simulink subsystem "PvtSubSys_LONC"  (R2020b)
settings: Solver=VariableStepAuto  StartTime=0.0  StopTime=10.0  RelTol=1e-3
undefined symbols (not defined in the file): P_Global_TireRadius_m, P_Global_Weight_N, P_LongCtrl_AxvRoadSlopeThrd, P_LongCtrl_SlideFlagEnable, P_LongCtrl_TotWheelTrqRatio, P_LongCtrl_VLC_fRollCoef, P_LongCtrl_VLC_WindArea, P_LongCtrl_VLCaccelMinHoldXAxis, P_LongCtrl_VLCaccelMinHoldYAxis, P_LongCtrl_VLCaccelMinSlidHoldXAxis, P_LongCtrl_VLCaccelMinSlidHoldYAxis, P_LongCtrl_VLCaDiffCharCoefKiEnableXAxis, P_LongCtrl_VLCaDiffCharCoefKiXAxis, P_LongCtrl_VLCaDtThresUpdateTorq, P_LongCtrl_VLCaXCDeadZoneProp_Y, P_LongCtrl_VLCaxCtrlDevDeadZoneChar_Y, P_LongCtrl_VLCaxCtrlDevEC2DCMax, P_LongCtrl_VLCaxCtrlDevFastQuitDCMode, P_LongCtrl_VLCaxCtrlDevThresAddEC2DCCharYAxis, P_LongCtrl_VLCaxCtrlDevTresAddDC2ECYAxis, P_LongCtrl_VLCaxDtCharAxCtrlDevTresAddDC2ECXAxis, P_LongCtrl_VLCaxDtCharAxCtrlDevTresAddEC2DCXAxis, P_LongCtrl_VLCAxTarDtThreEnableI, P_LongCtrl_VLCaxvRoadSlopeDC4CharXAxis, P_LongCtrl_VLCaxvRoadSlopeDC4CharYAxis, P_LongCtrl_VLCAxvTracMinDC1FullFillXAxis, P_LongCtrl_VLCAxvTracMinDC1FullFillYAxis, P_LongCtrl_VLCcoefFXAxis, P_LongCtrl_VLCcoefFYAxis, P_LongCtrl_VLCcoefIFadeOut1Calc, P_LongCtrl_VLCcoefIFadeOut1Condition, P_LongCtrl_VLCcoefIFadeOut2Calc, P_LongCtrl_VLCcoefIFadeOut2Condition, P_LongCtrl_VLCcoefIFadeOut3Calc, P_LongCtrl_VLCcoefIFadeOut3Condition, P_LongCtrl_VLCcoefKiDiffDtEnlargeYAxis, P_LongCtrl_VLCcoefKiEnableYAxis, P_LongCtrl_VLCcoefKiEnlargeADiffYAxis, P_LongCtrl_VLCcoefPIYAxis, P_LongCtrl_VLCCounterAxvTracMinTimeout, P_LongCtrl_VLCCounterDC2ECTorqDelay, P_LongCtrl_VLCCounterDrvOff2EC, P_LongCtrl_VLCdaxTarEC2DCMax, P_LongCtrl_VLCdiffDtCharCoefKiEnlargeXAxis, P_LongCtrl_VLCdriveOffAxUpLimXAxix, P_LongCtrl_VLCdriveOffAxUpLimYAxix, P_LongCtrl_VLCDtAxvRef2UpperBandDC5, P_LongCtrl_VLCengEfficientCharYAxis, P_LongCtrl_VLCengInverseEfficientYAxis, P_LongCtrl_VLCIACompensionNeg, P_LongCtrl_VLCIACompensionPos, P_LongCtrl_VLCjerkHoldXAxis, P_LongCtrl_VLCjerkHoldYAxis, P_LongCtrl_VLCjerkSlidHoldXAxis, P_LongCtrl_VLCjerkSlidHoldYAxis, P_LongCtrl_VLCki, P_LongCtrl_VLCkp, P_LongCtrl_VLCks, P_LongCtrl_VLCLowerJerkCounterDrvOff2EC, P_LongCtrl_VLCMaRatioCharMaYAxis ... (+12)
libraries: simulink x34
(part 2 of 3)

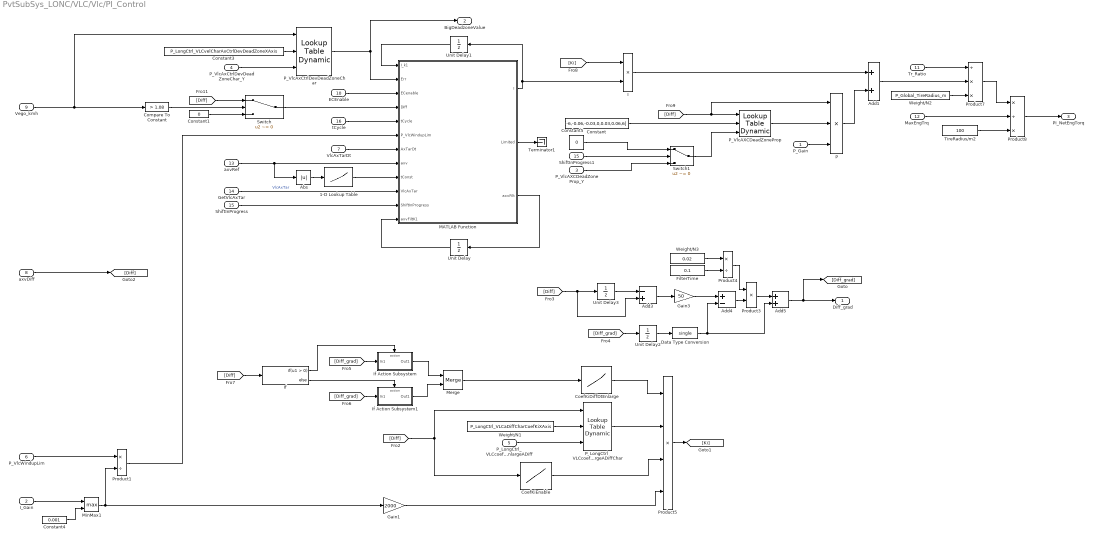
== system PvtSubSys_LONC/VLC/Vlc/PI_Control ==
  P_Gain : Inport
  I_Gain : Inport  Port=2
  P_VlcAXCDeadZoneProp_Y : Inport  Port=3
  P_VlcAxCtrlDevDeadZoneChar_Y : Inport  Port=4
  P_LongCtrl_VLCcoefKiEnlargeADiff : Inport  Port=5
  P_VlcWindupLim : Inport  Port=6
  VlcAxTarDt : Inport  Port=7
  axvDiff : Inport  Port=8
  Vego_kmh : Inport  Port=9
  ECEnable : Inport  Port=10
  Tr_Ratio : Inport  Port=11
  MaxEngTrq : Inport  Port=12
  axvRef : Inport  Port=13
  GetVlcAxTar : Inport  Port=14
  ShiftInProgress : Inport  Port=15
  tCycle : Inport  Port=16
  1-D Lookup Table : Lookup_n-D  NumberOfTableDimensions=1  BreakpointsForDimension1=[0,0.01,0.05,0.1,0.2,0.5]  Table=[0.02,0.06,0.1,0.2,0.3,0.3]  ExtrapMethod=Clip  UseLastTableValue=on  InternalRulePriority=Speed  RndMeth=Simplest  InputSameDT=on
  Abs : Abs
  Add1 : Sum
  Add3 : Sum  Inputs=-+
  Add4 : Sum  Inputs=+-  AccumDataTypeStr=single
  Add5 : Sum  AccumDataTypeStr=single
  CoefKiDiffDtEnlarge : Lookup_n-D  NumberOfTableDimensions=1  BreakpointsForDimension1=P_LongCtrl_VLCdiffDtCharCoefKiEnlargeXAxis  Table=P_LongCtrl_VLCcoefKiDiffDtEnlargeYAxis  ExtrapMethod=Clip  UseLastTableValue=on  RndMeth=Simplest  InputSameDT=on
  CoefKiEnable : Lookup_n-D  NumberOfTableDimensions=1  BreakpointsForDimension1=P_LongCtrl_VLCaDiffCharCoefKiEnableXAxis  Table=P_LongCtrl_VLCcoefKiEnableYAxis  ExtrapMethod=Clip  UseLastTableValue=on  RndMeth=Simplest  InputSameDT=on
  Compare To Constant : simulink/Logic and Bit Operations/Compare To Constant  relop=>  const=1.08  OutDataTypeStr=boolean
  Constant : Constant  Value=[-6,-0.06,-0.03,0,0.03,0.06,6]  OutDataTypeStr=single
  Constant1 : Constant  Value=0  OutDataTypeStr=single
  Constant3 : Constant  Description="0   36   72  108  120"  Value=P_LongCtrl_VLCvelCharAxCtrlDevDeadZoneXAxis  OutDataTypeStr=single
      settings: AttributesFormatString=%<Description>
  Constant4 : Constant  Value=0.001  OutDataTypeStr=single
  Constant5 : Constant  Value=0  OutDataTypeStr=single
  Data Type Conversion : DataTypeConversion  OutDataTypeStr=single
  FilterTime : Constant  Value=0.1  OutDataTypeStr=single
  Gain1 : Gain  Gain=2000
  Gain3 : Gain  Gain=50
  I : Product  RndMeth=Zero
  If : If
  If Action Subsystem : Subsystem  TreatAsAtomicUnit=on
  If Action Subsystem1 : Subsystem  TreatAsAtomicUnit=on
  MATLAB Function : MATLAB Function  TreatAsAtomicUnit=on
  Merge : Merge
  MinMax1 : MinMax  Function=max  Inputs=2
  P : Product  Inputs=3  RndMeth=Zero
  P_LongCtrl_VLCcoefKiEnlargeADiffChar : simulink/Lookup Tables/Lookup Table Dynamic  LookUpMeth=Interpolation-Use End Values  OutDataType=fixdt('single')  OutScaling=[]  OutputDataTypeScalingMode=Specify via dialog  OutDataTypeStr=single  DoSatur=off
  P_VlcAXCDeadZoneProp : simulink/Lookup Tables/Lookup Table Dynamic  LookUpMeth=Interpolation-Use End Values  OutDataType=fixdt('single')  OutScaling=[]  OutputDataTypeScalingMode=Specify via dialog  OutDataTypeStr=single  DoSatur=off
  P_VlcAxCtrlDevDeadZoneChar : simulink/Lookup Tables/Lookup Table Dynamic  LookUpMeth=Interpolation-Use End Values  OutDataType=fixdt('single')  OutScaling=[]  OutputDataTypeScalingMode=Specify via dialog  OutDataTypeStr=single  DoSatur=off
  Product1 : Product  Inputs=*/  RndMeth=Zero
  Product3 : Product  Inputs=**  RndMeth=Zero
  Product4 : Product  Inputs=*/  RndMeth=Zero
  Product5 : Product  Inputs=4  RndMeth=Zero
  Product7 : Product  Inputs=/**  RndMeth=Zero
  Product8 : Product  Inputs=*/*  RndMeth=Zero
  ShiftInProgress1 : InportShadow  Port=15
  Switch : Switch  Criteria=u2 ~= 0  Threshold=1.08
  Switch1 : Switch  Criteria=u2 ~= 0
  Terminator1 : Terminator
  TireRadius/m2 : Constant  Value=100  OutDataTypeStr=single
  Unit Delay : UnitDelay  SampleTime=-1  HasFrameUpgradeWarning=on
  Unit Delay1 : UnitDelay  SampleTime=-1  HasFrameUpgradeWarning=on
  Unit Delay2 : UnitDelay  InitialCondition=single(0)  SampleTime=-1  HasFrameUpgradeWarning=on
  Unit Delay3 : UnitDelay  SampleTime=-1  HasFrameUpgradeWarning=on
  Weight/N1 : Constant  Description="-2.5          -2        -0.4       -0.17        -0.1           0        0.15        0.25         0.6           3         3.5"  Value=P_LongCtrl_VLCaDiffCharCoefKiXAxis  OutDataTypeStr=single
      settings: AttributesFormatString=%<Description>
  Weight/N2 : Constant  Value=P_Global_TireRadius_m
  Weight/N3 : Constant  Value=0.02  OutDataTypeStr=single
  Diff_grad : Outport
  BigDeadzoneValue : Outport  Port=2
  PI_NetEngTorq : Outport  Port=3
  wires:
  Data Type Conversion/1 -> Add4/2, Add5/2
  Switch1/1 -> P_VlcAXCDeadZoneProp/3
  Constant5/1 -> Switch1/1
  ShiftInProgress1/1 -> Switch1/2
  Unit Delay/1 -> MATLAB Function/12(axvFiltK1)
  GetVlcAxTar/1 -> MATLAB Function/10(VlcAxTar)  "VlcAxTar"
  axvRef/1 -> Abs/1, MATLAB Function/8(axv)
  ShiftInProgress/1 -> MATLAB Function/11(ShiftInProgress)
  Abs/1 -> 1-D Lookup Table/1
  1-D Lookup Table/1 -> MATLAB Function/9(tConst)
  I_Gain/1 -> MinMax1/1
  Constant4/1 -> MinMax1/2
  axvDiff/1 -> [Diff]
  MATLAB Function/2(Limited) -> Terminator1/1
  Gain1/1 -> Product5/4
  Constant/1 -> P_VlcAXCDeadZoneProp/2
  MATLAB Function/3(axvFilt) -> Unit Delay/1
  Product1/1 -> MATLAB Function/6(P_VlcWindupLim)
  MinMax1/1 -> Product1/2, Gain1/1
  VlcAxTarDt/1 -> MATLAB Function/7(AxTarDt)
  P_VlcWindupLim/1 -> Product1/1
  I/1 -> Add1/1
  P_LongCtrl_VLCcoefKiEnlargeADiff/1 -> P_LongCtrl_VLCcoefKiEnlargeADiffChar/3
  Weight/N1/1 -> P_LongCtrl_VLCcoefKiEnlargeADiffChar/2
  Add1/1 -> Product7/2
  Product8/1 -> PI_NetEngTorq/1
  Weight/N2/1 -> Product7/3
  Tr_Ratio/1 -> Product7/1
  Product7/1 -> Product8/1
  MaxEngTrq/1 -> Product8/2
  TireRadius/m2/1 -> Product8/3
  P_VlcAxCtrlDevDeadZoneChar/1 -> MATLAB Function/2(Err), BigDeadzoneValue/1
  P_VlcAxCtrlDevDeadZoneChar_Y/1 -> P_VlcAxCtrlDevDeadZoneChar/3
  Constant3/1 -> P_VlcAxCtrlDevDeadZoneChar/2
  Unit Delay1/1 -> MATLAB Function/1(I_k1)
  ECEnable/1 -> MATLAB Function/3(ECenable)
  Switch/1 -> MATLAB Function/4(Diff)
  tCycle/1 -> MATLAB Function/5(tCycle)
  P_VlcAXCDeadZoneProp_Y/1 -> Switch1/3
  P_VlcAXCDeadZoneProp/1 -> P/2
  MATLAB Function/1(I) -> I/2, Unit Delay1/1
  [Diff] -> P_VlcAXCDeadZoneProp/1, P/1
  Product5/1 -> [Ki]
  CoefKiEnable/1 -> Product5/3
  P_LongCtrl_VLCcoefKiEnlargeADiffChar/1 -> Product5/2
  CoefKiDiffDtEnlarge/1 -> Product5/1
  [Diff] -> CoefKiEnable/1, P_LongCtrl_VLCcoefKiEnlargeADiffChar/1
  FilterTime/1 -> Product4/2
  Product4/1 -> Product3/1
  Weight/N3/1 -> Product4/1
  [Diff] -> If/1
  Merge/1 -> CoefKiDiffDtEnlarge/1
  If Action Subsystem1/1(Out1) -> Merge/2
  If Action Subsystem/1(Out1) -> Merge/1
  [Diff_grad] -> If Action Subsystem1/1(In1)
  [Diff_grad] -> If Action Subsystem/1(In1)
  If/2 -> If Action Subsystem1/Action
  If/1 -> If Action Subsystem/Action
  [Diff] -> Add3/2, Unit Delay3/1
  Gain3/1 -> Add4/1
  Add5/1 -> Diff_grad/1, [Diff_grad]
  Product3/1 -> Add5/1
  Add4/1 -> Product3/2
  Add3/1 -> Gain3/1
  Unit Delay2/1 -> Data Type Conversion/1
  [Diff_grad] -> Unit Delay2/1
  Unit Delay3/1 -> Add3/1
  Constant1/1 -> Switch/3
  Vego_kmh/1 -> P_VlcAxCtrlDevDeadZoneChar/1, Compare To Constant/1
  [Diff] -> Switch/1
  [Ki] -> I/1
  P/1 -> Add1/2
  P_Gain/1 -> P/3
  Compare To Constant/1 -> Switch/2

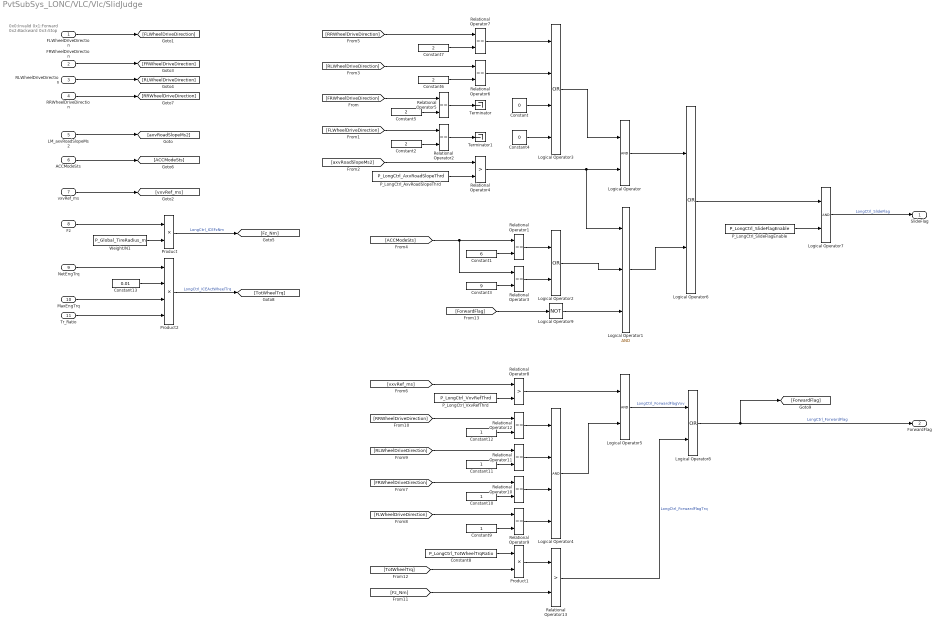
== system PvtSubSys_LONC/VLC/Vlc/SlidJudge ==
  note: 0x0:Invalid
      | 0x1:Forward
      | 0x2:Backward
      | 0x3:Stop
  FLWheelDriveDirection : Inport
  FRWheelDriveDirection : Inport  Port=2
  RLWheelDriveDirection : Inport  Port=3
  RRWheelDriveDirection : Inport  Port=4
  LM_axvRoadSlopeMs2 : Inport  Port=5
  ACCModeSts : Inport  Port=6
  vxvRef_ms : Inport  Port=7
  Fz : Inport  Port=8
  NetEngTrq : Inport  Port=9
  MaxEngTrq : Inport  Port=10
  Tr_Ratio : Inport  Port=11
  Constant : Constant  Value=0  OutDataTypeStr=boolean
  Constant1 : Constant  Value=6
  Constant{9..12} (4 alike) : Constant
  Constant13 : Constant  Value=0.01
  Constant{2,5..7} (4 alike) : Constant  Value=2
  Constant3 : Constant  Value=9
  Constant4 : Constant  Value=0  OutDataTypeStr=boolean
  Constant8 : Constant  Value=P_LongCtrl_TotWheelTrqRatio
  Logical Operator : Logic  AllPortsSameDT=off  OutDataTypeStr=boolean
  Logical Operator1 : Logic  Inputs=3  AllPortsSameDT=off  OutDataTypeStr=boolean
  Logical Operator2 : Logic  Operator=OR  AllPortsSameDT=off  OutDataTypeStr=boolean
  Logical Operator3 : Logic  Operator=OR  Inputs=4  AllPortsSameDT=off  OutDataTypeStr=boolean
  Logical Operator4 : Logic  Inputs=4  AllPortsSameDT=off  OutDataTypeStr=boolean
  Logical Operator5 : Logic  AllPortsSameDT=off  OutDataTypeStr=boolean
  Logical Operator6 : Logic  Operator=OR  AllPortsSameDT=off  OutDataTypeStr=boolean
  Logical Operator7 : Logic  AllPortsSameDT=off  OutDataTypeStr=boolean
  Logical Operator8 : Logic  Operator=OR  AllPortsSameDT=off  OutDataTypeStr=boolean
  Logical Operator9 : Logic  Operator=NOT  AllPortsSameDT=off  OutDataTypeStr=boolean
  P_LongCtrl_AxvRoadSlopeThrd : Constant  Description=0.1  Value=P_LongCtrl_AxvRoadSlopeThrd
      settings: AttributesFormatString=%<Description>
  P_LongCtrl_SlideFlagEnable : Constant  Description=0  Value=P_LongCtrl_SlideFlagEnable
      settings: AttributesFormatString=%<Description>
  P_LongCtrl_VxvRefThrd : Constant  Description=0.1  Value=P_LongCtrl_VxvRefThrd
      settings: AttributesFormatString=%<Description>
  Product : Product
  Product1 : Product
  Product2 : Product  Inputs=4
  Relational Operator{1..3,5..7,9..12} (10 alike) : RelationalOperator  Operator===  OutDataTypeStr=boolean  RndMeth=Simplest
  Relational Operator13 : RelationalOperator  Operator=>  OutDataTypeStr=boolean  RndMeth=Simplest
  Relational Operator4 : RelationalOperator  Operator=>  OutDataTypeStr=boolean  RndMeth=Simplest
  Relational Operator8 : RelationalOperator  Operator=>  OutDataTypeStr=boolean  RndMeth=Simplest
  Terminator : Terminator
  Terminator1 : Terminator
  Weight/N1 : Constant  Value=P_Global_TireRadius_m
  SlideFlag : Outport
  ForwardFlag : Outport  Port=2
  wires:
  Constant2/1 -> Relational Operator2/2
  FRWheelDriveDirection/1 -> [FRWheelDriveDirection]
  RLWheelDriveDirection/1 -> [RLWheelDriveDirection]
  RRWheelDriveDirection/1 -> [RRWheelDriveDirection]
  LM_axvRoadSlopeMs2/1 -> [axvRoadSlopeMs2]
  P_LongCtrl_AxvRoadSlopeThrd/1 -> Relational Operator4/2
  Relational Operator2/1 -> Terminator1/1
  Relational Operator4/1 -> Logical Operator1/1, Logical Operator/2
  FLWheelDriveDirection/1 -> [FLWheelDriveDirection]
  [FLWheelDriveDirection] -> Relational Operator2/1
  [axvRoadSlopeMs2] -> Relational Operator4/1
  ACCModeSts/1 -> [ACCModeSts]
  [ACCModeSts] -> Relational Operator3/1, Relational Operator1/1
  Constant1/1 -> Relational Operator1/2
  Constant3/1 -> Relational Operator3/2
  Relational Operator1/1 -> Logical Operator2/1
  Relational Operator3/1 -> Logical Operator2/2
  Logical Operator2/1 -> Logical Operator1/2
  Logical Operator1/1 -> Logical Operator6/2
  Logical Operator/1 -> Logical Operator6/1
  Relational Operator5/1 -> Terminator/1
  Constant5/1 -> Relational Operator5/2
  Constant6/1 -> Relational Operator6/2
  Relational Operator6/1 -> Logical Operator3/2
  Relational Operator7/1 -> Logical Operator3/1
  Constant7/1 -> Relational Operator7/2
  [RRWheelDriveDirection] -> Relational Operator7/1
  [RLWheelDriveDirection] -> Relational Operator6/1
  [FRWheelDriveDirection] -> Relational Operator5/1
  Logical Operator3/1 -> Logical Operator/1
  vxvRef_ms/1 -> [vxvRef_ms]
  [vxvRef_ms] -> Relational Operator8/1
  P_LongCtrl_VxvRefThrd/1 -> Relational Operator8/2
  [FRWheelDriveDirection] -> Relational Operator10/1
  [RLWheelDriveDirection] -> Relational Operator11/1
  [RRWheelDriveDirection] -> Relational Operator12/1
  Constant12/1 -> Relational Operator12/2
  Relational Operator12/1 -> Logical Operator4/1
  Relational Operator11/1 -> Logical Operator4/2
  Constant11/1 -> Relational Operator11/2
  Constant10/1 -> Relational Operator10/2
  Relational Operator10/1 -> Logical Operator4/3
  [FLWheelDriveDirection] -> Relational Operator9/1
  Relational Operator9/1 -> Logical Operator4/4
  Constant9/1 -> Relational Operator9/2
  Relational Operator8/1 -> Logical Operator5/1
  Logical Operator4/1 -> Logical Operator5/2
  Logical Operator5/1 -> Logical Operator8/1  "LongCtrl_ForwardFlagVxv"
  Logical Operator6/1 -> Logical Operator7/1
  Logical Operator7/1 -> SlideFlag/1  "LongCtrl_SlideFlag"
  P_LongCtrl_SlideFlagEnable/1 -> Logical Operator7/2
  Constant/1 -> Logical Operator3/3
  Constant4/1 -> Logical Operator3/4
  Fz/1 -> Product/1
  Weight/N1/1 -> Product/2
  Product/1 -> [Fz_Nm]  "LongCtrl_ICEFzNm"
  NetEngTrq/1 -> Product2/1
  [TotWheelTrq] -> Product1/2
  Product1/1 -> Relational Operator13/1
  [Fz_Nm] -> Relational Operator13/2
  Constant8/1 -> Product1/1
  Logical Operator8/1 -> [ForwardFlag], ForwardFlag/1  "LongCtrl_ForwardFlag"
  Relational Operator13/1 -> Logical Operator8/2  "LongCtrl_ForwardFlagTrq"
  MaxEngTrq/1 -> Product2/3
  Constant13/1 -> Product2/2
  Tr_Ratio/1 -> Product2/4
  Product2/1 -> [TotWheelTrq]  "LongCtrl_ICEActWheelTrq"
  [ForwardFlag] -> Logical Operator9/1
  Logical Operator9/1 -> Logical Operator1/3

== system PvtSubSys_LONC/VLC/Vlc/Subsystem ==
  u : Inport
  MATLAB Function : MATLAB Function  TreatAsAtomicUnit=on
  Tapped Delay2 : simulink/Discrete/Tapped Delay  vinit=0.0  samptime=-1  NumDelays=1  DelayOrder=Newest  includeCurrent=on
  Unit Delay : UnitDelay  SampleTime=-1  HasFrameUpgradeWarning=on
  ACCModeSts : Outport
  wires:
  MATLAB Function/1(ACCModeSts) -> ACCModeSts/1
  u/1 -> Tapped Delay2/1
  Tapped Delay2/1 -> MATLAB Function/1(u)
  MATLAB Function/2(CounterK1) -> Unit Delay/1
  Unit Delay/1 -> MATLAB Function/2(Counter)

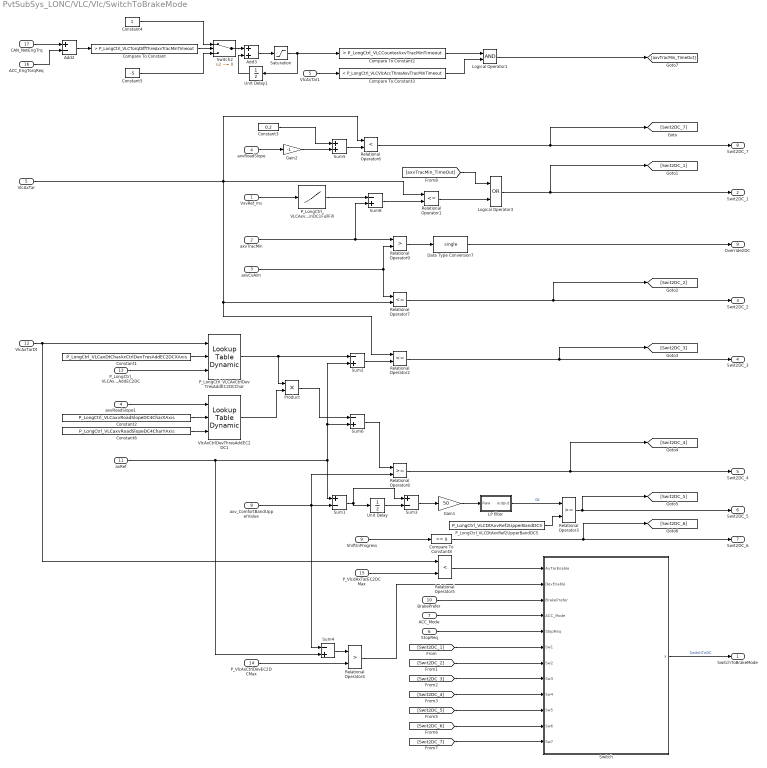
== system PvtSubSys_LONC/VLC/Vlc/SwitchToBrakeMode ==
  VxvRef_ms : Inport
  axvTracMin : Inport  Port=2
  axvCvAim : Inport  Port=3
  axvRoadSlope : Inport  Port=4
  VlcAxTar : Inport  Port=5
  StopReq : Inport  Port=6
  ACC_Mode : Inport  Port=7  OutDataTypeStr=uint8
  axv_ComfortBandUpperValue : Inport  Port=8
  "ShiftInProgress " : Inport  Port=9
  BrakePrefer : Inport  Port=10
  axRef : Inport  Port=11
  VlcAxTarDt : Inport  Port=12
  P_LongCtrl_VLCAxCtrlDevTresAddEC2DC : Inport  Port=13
  P_VlcAxCtrlDevEC2DCMax : Inport  Port=14
  P_VlcdAxTarEC2DCMax : Inport  Port=15
  ACC_EngTorqReq : Inport  Port=16  OutDataTypeStr=single
  CAN_NetEngTrq : Inport  Port=17  OutDataTypeStr=single
  Add2 : Sum  Inputs=+-
  Add3 : Sum  AccumDataTypeStr=single
  Compare To Constant : simulink/Logic and Bit Operations/Compare To Constant  Description=4  relop=>  const=P_LongCtrl_VLCTorqDiffThreAxvTracMinTimeout  OutDataTypeStr=boolean
      settings: AttributesFormatString=%<Description>
  Compare To Constant2 : simulink/Logic and Bit Operations/Compare To Constant  Description=40  relop=>  const=P_LongCtrl_VLCCounterAxvTracMinTimeout  OutDataTypeStr=boolean
      settings: AttributesFormatString=%<Description>
  Compare To Constant3 : simulink/Logic and Bit Operations/Compare To Constant  Description=0  relop=<  const=P_LongCtrl_VLCVlcAccThresAxvTracMinTimeout  OutDataTypeStr=boolean
      settings: AttributesFormatString=%<Description>
  Compare To Constant8 : simulink/Logic and Bit Operations/Compare To Constant  relop===  const=0  OutDataTypeStr=boolean
  Constant1 : Constant  Description="-0.7        -0.5        -0.3        -0.1           0"  Value=P_LongCtrl_VLCaxDtCharAxCtrlDevTresAddEC2DCXAxis  OutDataTypeStr=single
      settings: AttributesFormatString=%<Description>
  Constant2 : Constant  Description="-0.5        -0.3        -0.2        -0.1           0"  Value=P_LongCtrl_VLCaxvRoadSlopeDC4CharXAxis  OutDataTypeStr=single
      settings: AttributesFormatString=%<Description>
  Constant3 : Constant  Value=0.2  OutDataTypeStr=single
  Constant4 : Constant  OutDataTypeStr=single
  Constant5 : Constant  Value=-5  OutDataTypeStr=single
  Constant6 : Constant  Description="0         0.2         0.4         0.8           1"  Value=P_LongCtrl_VLCaxvRoadSlopeDC4CharYAxis  OutDataTypeStr=single
      settings: AttributesFormatString=%<Description>
  Data Type Conversion7 : DataTypeConversion  OutDataTypeStr=single
  Gain1 : Gain  Gain=50
  Gain2 : Gain  Gain=-1
  LP filter : Subsystem
  Logical Operator1 : Logic  AllPortsSameDT=off  OutDataTypeStr=boolean
  Logical Operator3 : Logic  Operator=OR  AllPortsSameDT=off  OutDataTypeStr=boolean
  P_LongCtrl_VLCAxCtrlDevTresAddEC2DCChar : simulink/Lookup Tables/Lookup Table Dynamic  LookUpMeth=Interpolation-Use End Values  OutDataType=fixdt('single')  OutScaling=[]  OutputDataTypeScalingMode=Specify via dialog  OutDataTypeStr=single  DoSatur=off
  P_LongCtrl_VLCAxvTracMinDC1FullFill : Lookup_n-D  NumberOfTableDimensions=1  BreakpointsForDimension1=P_LongCtrl_VLCAxvTracMinDC1FullFillXAxis  Table=P_LongCtrl_VLCAxvTracMinDC1FullFillYAxis  ExtrapMethod=Clip  UseLastTableValue=on  RndMeth=Simplest  InputSameDT=on
  P_LongCtrl_VLCDtAxvRef2UpperBandDC5 : Constant  Description=-0.5  Value=P_LongCtrl_VLCDtAxvRef2UpperBandDC5  OutDataTypeStr=single
      settings: AttributesFormatString=%<Description>
  Product : Product
  Relational Operator1 : RelationalOperator  Operator=<=  OutDataTypeStr=boolean  RndMeth=Nearest
  Relational Operator2 : RelationalOperator  Operator=<=  OutDataTypeStr=boolean  RndMeth=Nearest
  Relational Operator3 : RelationalOperator  OutDataTypeStr=boolean  RndMeth=Nearest
  Relational Operator4 : RelationalOperator  Operator=>  OutDataTypeStr=boolean  RndMeth=Nearest
  Relational Operator5 : RelationalOperator  Operator=<  OutDataTypeStr=boolean  RndMeth=Nearest
  Relational Operator6 : RelationalOperator  Operator=<  OutDataTypeStr=boolean  RndMeth=Nearest
  Relational Operator7 : RelationalOperator  Operator=<=  OutDataTypeStr=boolean  RndMeth=Nearest
  Relational Operator8 : RelationalOperator  OutDataTypeStr=boolean  RndMeth=Nearest
  Relational Operator9 : RelationalOperator  Operator=>  OutDataTypeStr=boolean  RndMeth=Nearest
  Saturation : Saturate  UpperLimit=100  LowerLimit=0  OutDataTypeStr=single
  Sum1 : Sum  Inputs=+-
  Sum{2,4,6,8} (4 alike) : Sum  Inputs=-+
  Sum3 : Sum  Inputs=+-
  Sum5 : Sum
  Switch : MATLAB Function  TreatAsAtomicUnit=on
  Switch2 : Switch  Criteria=u2 ~= 0  Threshold=P_LongCtrl_VLCTorqDiffThreAxvTracMinTimeout
  Unit Delay : UnitDelay  SampleTime=-1  HasFrameUpgradeWarning=on
  Unit Delay1 : UnitDelay  SampleTime=-1  HasFrameUpgradeWarning=on
  VlcAxCtrlDevThresAddEC2DC1 : simulink/Lookup Tables/Lookup Table Dynamic  LookUpMeth=Interpolation-Use End Values  OutDataType=fixdt('single')  OutScaling=[]  OutputDataTypeScalingMode=Specify via dialog  OutDataTypeStr=single  DoSatur=off
  VlcAxTar1 : InportShadow  Port=5
  axvRoadSlope1 : InportShadow  Port=4
  SwitchToBrakeMode : Outport
  Swit2DC_1 : Outport  Port=2
  Swit2DC_2 : Outport  Port=3
  Swit2DC_3 : Outport  Port=4
  Swit2DC_4 : Outport  Port=5
  Swit2DC_5 : Outport  Port=6
  Swit2DC_6 : Outport  Port=7
  Swit2DC_7 : Outport  Port=8
  Override2DC : Outport  Port=9
  wires:
  Product/1 -> Sum6/1
  Constant6/1 -> VlcAxCtrlDevThresAddEC2DC1/3
  axvRoadSlope1/1 -> VlcAxCtrlDevThresAddEC2DC1/1
  VlcAxCtrlDevThresAddEC2DC1/1 -> Product/2
  P_LongCtrl_VLCAxCtrlDevTresAddEC2DCChar/1 -> Product/1, Sum2/1
  Constant2/1 -> VlcAxCtrlDevThresAddEC2DC1/2
  Sum6/1 -> Relational Operator8/1
  Saturation/1 -> Unit Delay1/1, Compare To Constant2/1
  Relational Operator1/1 -> Logical Operator3/2
  [axvTracMin_TimeOut] -> Logical Operator3/1
  Logical Operator1/1 -> [axvTracMin_TimeOut]
  VlcAxTar1/1 -> Compare To Constant3/1
  ACC_EngTorqReq/1 -> Add2/2
  CAN_NetEngTrq/1 -> Add2/1
  Switch2/1 -> Add3/1
  Constant5/1 -> Switch2/3
  Compare To Constant3/1 -> Logical Operator1/2
  Compare To Constant2/1 -> Logical Operator1/1
  Add3/1 -> Saturation/1
  Unit Delay1/1 -> Add3/2
  Constant4/1 -> Switch2/1
  Data Type Conversion7/1 -> Override2DC/1
  Relational Operator9/1 -> Data Type Conversion7/1
  axvCvAim/1 -> Relational Operator9/2, Relational Operator7/1
  [Swit2DC_1] -> Switch/6(Sw1)
  [Swit2DC_2] -> Switch/7(Sw2)
  [Swit2DC_3] -> Switch/8(Sw3)
  [Swit2DC_4] -> Switch/9(Sw4)
  [Swit2DC_5] -> Switch/10(Sw5)
  [Swit2DC_6] -> Switch/11(Sw6)
  [Swit2DC_7] -> Switch/12(Sw7)
  StopReq/1 -> Switch/5(StopReq)
  ACC_Mode/1 -> Switch/4(ACC_Mode)
  BrakePrefer/1 -> Switch/3(BrakePrefer)
  Relational Operator4/1 -> Switch/2(DevEnable)
  Relational Operator5/1 -> Switch/1(AxTarEnable)
  Compare To Constant8/1 -> Swit2DC_6/1, [Swit2DC_6]
  "ShiftInProgress "/1 -> Compare To Constant8/1
  Relational Operator3/1 -> Swit2DC_5/1, [Swit2DC_5]
  Relational Operator8/1 -> [Swit2DC_4], Swit2DC_4/1
  Relational Operator2/1 -> [Swit2DC_3], Swit2DC_3/1
  Relational Operator7/1 -> [Swit2DC_2], Swit2DC_2/1
  Logical Operator3/1 -> [Swit2DC_1], Swit2DC_1/1
  Relational Operator6/1 -> [Swit2DC_7], Swit2DC_7/1
  Sum5/1 -> Relational Operator6/2
  VlcAxTar/1 -> Relational Operator6/1, Relational Operator1/1, Relational Operator2/1, Relational Operator7/2
  Constant3/1 -> Sum5/1
  Gain2/1 -> Sum5/2
  axvRoadSlope/1 -> Gain2/1
  P_LongCtrl_VLCAxvTracMinDC1FullFill/1 -> Sum8/1
  P_VlcdAxTarEC2DCMax/1 -> Relational Operator5/2
  P_VlcAxCtrlDevEC2DCMax/1 -> Relational Operator4/2
  Sum4/1 -> Relational Operator4/1
  axv_ComfortBandUpperValue/1 -> Sum4/1, Relational Operator8/2, Sum1/2
  P_LongCtrl_VLCDtAxvRef2UpperBandDC5/1 -> Relational Operator3/2
  P_LongCtrl_VLCAxCtrlDevTresAddEC2DC/1 -> P_LongCtrl_VLCAxCtrlDevTresAddEC2DCChar/3
  Constant1/1 -> P_LongCtrl_VLCAxCtrlDevTresAddEC2DCChar/2
  VlcAxTarDt/1 -> Relational Operator5/1, P_LongCtrl_VLCAxCtrlDevTresAddEC2DCChar/1
  LP filter/1(output) -> Relational Operator3/1  "Dt"
  Gain1/1 -> LP filter/1(Raw)
  Sum3/1 -> Gain1/1
  Unit Delay/1 -> Sum3/2
  Sum2/1 -> Relational Operator2/2
  Sum1/1 -> Unit Delay/1, Sum3/1
  axRef/1 -> Sum1/1, Sum2/2, Sum6/2, Sum4/2
  Switch/1(y) -> SwitchToBrakeMode/1  "SwitchToDC"
  Sum8/1 -> Relational Operator1/2
  axvTracMin/1 -> Sum8/2, Relational Operator9/1
  VxvRef_ms/1 -> P_LongCtrl_VLCAxvTracMinDC1FullFill/1
  Add2/1 -> Compare To Constant/1
  Compare To Constant/1 -> Switch2/2

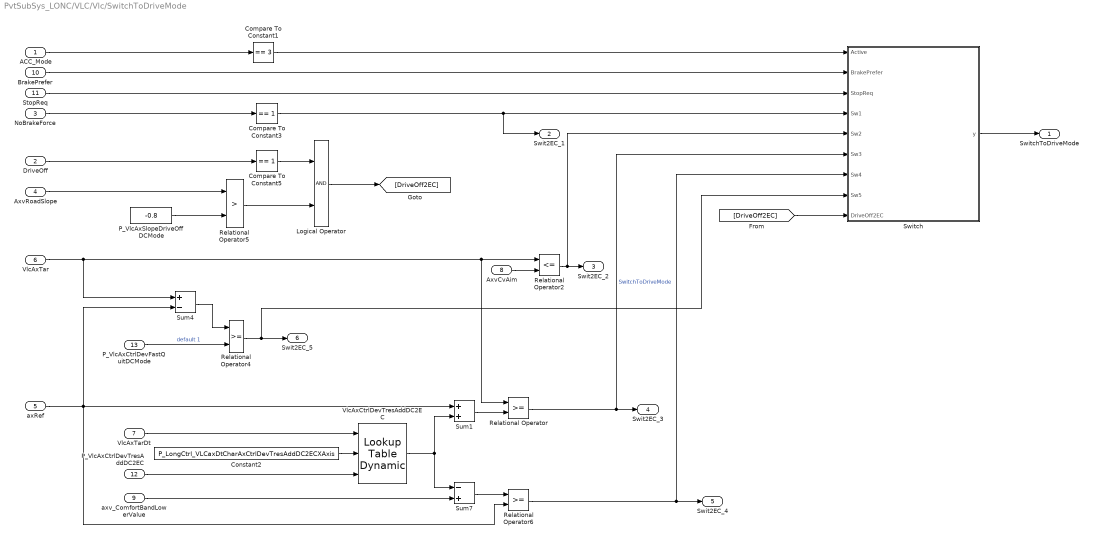
== system PvtSubSys_LONC/VLC/Vlc/SwitchToDriveMode ==
  ACC_Mode : Inport
  DriveOff : Inport  Port=2
  NoBrakeForce : Inport  Port=3
  AxvRoadSlope : Inport  Port=4
  axRef : Inport  Port=5
  VlcAxTar : Inport  Port=6
  VlcAxTarDt : Inport  Port=7
  AxvCvAim : Inport  Port=8
  axv_ComfortBandLowerValue : Inport  Port=9
  BrakePrefer : Inport  Port=10
  StopReq : Inport  Port=11
  P_VlcAxCtrlDevTresAddDC2EC : Inport  Port=12
  P_VlcAxCtrlDevFastQuitDCMode : Inport  Port=13
  Compare To Constant1 : simulink/Logic and Bit Operations/Compare To Constant  relop===  const=3  OutDataTypeStr=boolean
  Compare To Constant3 : simulink/Logic and Bit Operations/Compare To Constant  relop===  const=1  OutDataTypeStr=boolean
  Compare To Constant5 : simulink/Logic and Bit Operations/Compare To Constant  relop===  const=1  OutDataTypeStr=boolean
  Constant2 : Constant  Description="0         0.1         0.3         0.5         0.7"  Value=P_LongCtrl_VLCaxDtCharAxCtrlDevTresAddDC2ECXAxis  OutDataTypeStr=single
      settings: AttributesFormatString=%<Description>
  Logical Operator : Logic  AllPortsSameDT=off  OutDataTypeStr=boolean
  P_VlcAxSlopeDriveOffDCMode : Constant  Value=-0.8
  Relational Operator : RelationalOperator  OutDataTypeStr=boolean  RndMeth=Nearest
  Relational Operator2 : RelationalOperator  Operator=<=  OutDataTypeStr=boolean  RndMeth=Nearest
  Relational Operator4 : RelationalOperator  OutDataTypeStr=boolean  RndMeth=Nearest
  Relational Operator5 : RelationalOperator  Operator=>  OutDataTypeStr=boolean  RndMeth=Nearest
  Relational Operator6 : RelationalOperator  OutDataTypeStr=boolean  RndMeth=Nearest
  Sum1 : Sum
  Sum4 : Sum  Inputs=+-
  Sum7 : Sum  Inputs=-+
  Switch : MATLAB Function  TreatAsAtomicUnit=on
  VlcAxCtrlDevTresAddDC2EC : simulink/Lookup Tables/Lookup Table Dynamic  LookUpMeth=Interpolation-Use End Values  OutDataType=fixdt('double')  OutScaling=[]  OutputDataTypeScalingMode=Specify via dialog  OutDataTypeStr=fixdt('double')  DoSatur=off
  SwitchToDriveMode : Outport
  Swit2EC_1 : Outport  Port=2
  Swit2EC_2 : Outport  Port=3
  Swit2EC_3 : Outport  Port=4
  Swit2EC_4 : Outport  Port=5
  Swit2EC_5 : Outport  Port=6
  wires:
  StopReq/1 -> Switch/3(StopReq)
  [DriveOff2EC] -> Switch/9(DriveOff2EC)
  Compare To Constant3/1 -> Switch/4(Sw1), Swit2EC_1/1
  Relational Operator2/1 -> Swit2EC_2/1, Switch/5(Sw2)
  Relational Operator6/1 -> Swit2EC_4/1, Switch/7(Sw4)
  Relational Operator4/1 -> Swit2EC_5/1, Switch/8(Sw5)
  BrakePrefer/1 -> Switch/2(BrakePrefer)
  Sum4/1 -> Relational Operator4/1
  axv_ComfortBandLowerValue/1 -> Sum7/2
  Relational Operator/1 -> Swit2EC_3/1, Switch/6(Sw3)  "SwitchToDriveMode"
  Sum7/1 -> Relational Operator6/1
  Sum1/1 -> Relational Operator/2
  AxvCvAim/1 -> Relational Operator2/2
  VlcAxTar/1 -> Relational Operator2/1, Relational Operator/1, Sum4/1
  Relational Operator5/1 -> Logical Operator/2
  P_VlcAxSlopeDriveOffDCMode/1 -> Relational Operator5/2
  AxvRoadSlope/1 -> Relational Operator5/1
  Switch/1(y) -> SwitchToDriveMode/1
  P_VlcAxCtrlDevFastQuitDCMode/1 -> Relational Operator4/2  "default 1"
  axRef/1 -> Sum4/2, Relational Operator6/2, Sum1/1
  Compare To Constant1/1 -> Switch/1(Active)
  Logical Operator/1 -> [DriveOff2EC]
  Compare To Constant5/1 -> Logical Operator/1
  DriveOff/1 -> Compare To Constant5/1
  ACC_Mode/1 -> Compare To Constant1/1
  VlcAxCtrlDevTresAddDC2EC/1 -> Sum1/2, Sum7/1
  P_VlcAxCtrlDevTresAddDC2EC/1 -> VlcAxCtrlDevTresAddDC2EC/3
  Constant2/1 -> VlcAxCtrlDevTresAddDC2EC/2
  VlcAxTarDt/1 -> VlcAxCtrlDevTresAddDC2EC/1
  NoBrakeForce/1 -> Compare To Constant3/1

== system PvtSubSys_LONC/VLC/Vlc/UpdateFlagCalc ==
  NoBrakeForce : Inport
  DCT_ShiftInProgress : Inport  Port=2
  AxRefDt : Inport  Port=3
  Vxv : Inport  Port=4
  Abs4 : Abs
  Compare To Constant1 : simulink/Logic and Bit Operations/Compare To Constant  Description=5  relop=<=  const=P_LongCtrl_VLCaDtThresUpdateTorq  OutDataTypeStr=boolean
      settings: AttributesFormatString=%<Description>
  Compare To Constant2 : simulink/Logic and Bit Operations/Compare To Constant  Description=18  relop=>=  const=P_LongCtrl_VLCvelThresUpdateTorq  OutDataTypeStr=boolean
      settings: AttributesFormatString=%<Description>
  Compare To Constant4 : simulink/Logic and Bit Operations/Compare To Constant  relop===  const=0  OutDataTypeStr=boolean
  Compare To Constant7 : simulink/Logic and Bit Operations/Compare To Constant  relop===  const=6  OutDataTypeStr=boolean
  Compare To Constant8 : simulink/Logic and Bit Operations/Compare To Constant  relop===  const=0  OutDataTypeStr=boolean
  Logical Operator : Logic  Inputs=5  AllPortsSameDT=off  OutDataTypeStr=boolean
  Sum of Elements1 : Sum  Inputs=+
  Tapped Delay1 : simulink/Discrete/Tapped Delay  vinit=0.0  samptime=-1  NumDelays=5  DelayOrder=Newest  includeCurrent=on
  Timer : Subsystem
  UpdateEnable : Outport
  wires:
  Vxv/1 -> Compare To Constant2/1
  Compare To Constant1/1 -> Logical Operator/2
  Logical Operator/1 -> UpdateEnable/1
  NoBrakeForce/1 -> Tapped Delay1/1
  Timer/1(Timer) -> Compare To Constant4/1
  Compare To Constant7/1 -> Logical Operator/1
  Compare To Constant4/1 -> Logical Operator/5
  DCT_ShiftInProgress/1 -> Compare To Constant8/1, Timer/1(Falling)
  AxRefDt/1 -> Abs4/1
  Tapped Delay1/1 -> Sum of Elements1/1
  Sum of Elements1/1 -> Compare To Constant7/1
  Compare To Constant2/1 -> Logical Operator/3
  Compare To Constant8/1 -> Logical Operator/4
  Abs4/1 -> Compare To Constant1/1

== system PvtSubSys_LONC/VLC/Vlc/axvClosedLoopControlCalc ==
  axvModelResidual : Inport
  VlcInternalAcc : Inport  Port=2
  AxRef : Inport  Port=3
  Abs : Abs
  Abs1 : Abs
  Constant : Constant  Value=0.02  OutDataTypeStr=single
  Constant1 : Constant  Value=0.02  OutDataTypeStr=single
  LP1 : Subsystem
  MinMax : MinMax  Inputs=2
  Product : Product  Inputs=*/  RndMeth=Zero
  Product1 : Product  Inputs=*/  RndMeth=Zero
  Sum3 : Sum
  Sum4 : Sum  Inputs=+-
  Sum5 : Sum  Inputs=+-
  Unit Delay : UnitDelay  SampleTime=-1  HasFrameUpgradeWarning=on
  "tfxvCvFilter1 " : Lookup_n-D  NumberOfTableDimensions=1  BreakpointsForDimension1=[0,0.1,0.2,1]  Table=[0.1,0.1,0.04,0.04]  ExtrapMethod=Clip  UseLastTableValue=on  RndMeth=Simplest  InputSameDT=on
  tfxvCvFilter2 : Lookup_n-D  NumberOfTableDimensions=1  BreakpointsForDimension1=[0,0.1,0.2,1]  Table=[0.1,0.1,0.02,0.02]  ExtrapMethod=Clip  UseLastTableValue=on  RndMeth=Simplest  InputSameDT=on
  axvClosedLoopControl : Outport
  tauFxvCvFilter : Outport  Port=2
  Diff : Outport  Port=3
  wires:
  AxRef/1 -> Sum5/2
  LP1/1(Out) -> Abs/1
  axvModelResidual/1 -> Sum3/1
  MinMax/1 -> tauFxvCvFilter/1
  Product1/1 -> MinMax/2
  Product/1 -> MinMax/1
  tfxvCvFilter2/1 -> Product1/2
  Constant1/1 -> Product1/1
  "tfxvCvFilter1 "/1 -> Product/2
  Constant/1 -> Product/1
  Abs1/1 -> tfxvCvFilter2/1
  Sum5/1 -> Diff/1, Abs1/1
  VlcInternalAcc/1 -> Sum3/2, Sum5/1
  [aDtxvCvABS] -> "tfxvCvFilter1 "/1
  Abs/1 -> [aDtxvCvABS]
  Sum4/1 -> LP1/1(Raw)
  Unit Delay/1 -> Sum4/2
  Sum3/1 -> axvClosedLoopControl/1, Sum4/1, Unit Delay/1

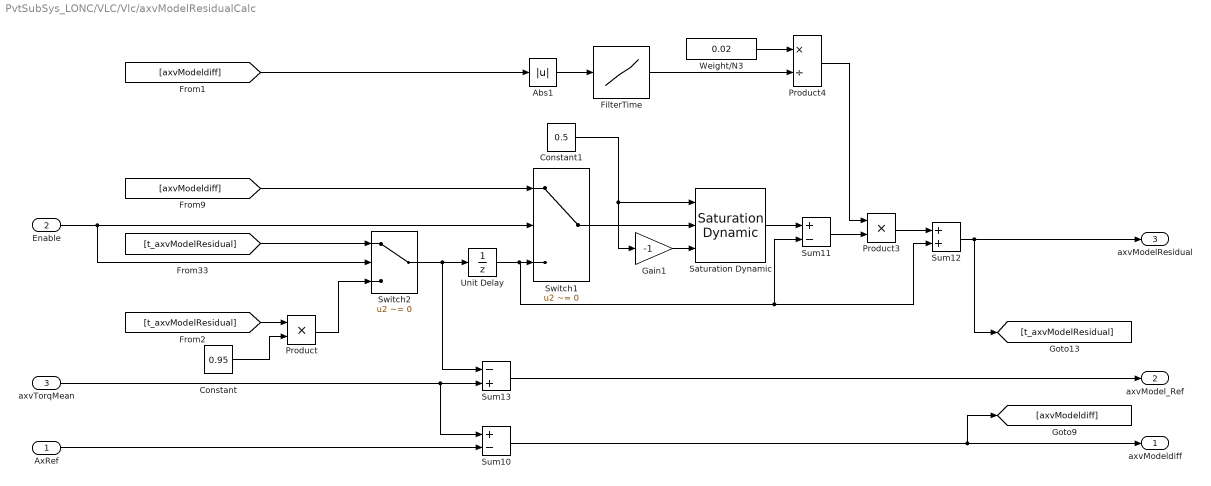
== system PvtSubSys_LONC/VLC/Vlc/axvModelResidualCalc ==
  AxRef : Inport
  Enable : Inport  Port=2
  axvTorqMean : Inport  Port=3
  Abs1 : Abs
  Constant : Constant  Value=0.95  OutDataTypeStr=single
  Constant1 : Constant  Value=0.5  OutDataTypeStr=single
  FilterTime : Lookup_n-D  NumberOfTableDimensions=1  BreakpointsForDimension1=[0,0.1,0.4,0.8,1]  Table=[1,0.4,0.1,0.04,0.04]  ExtrapMethod=Clip  UseLastTableValue=on  RndMeth=Simplest  InputSameDT=on
  Gain1 : Gain  Gain=-1
  Product : Product  OutDataTypeStr=single
  Product3 : Product  RndMeth=Zero
  Product4 : Product  Inputs=*/  RndMeth=Zero
  Saturation Dynamic : simulink/Discontinuities/Saturation Dynamic  OutMin=[]  OutMax=[]  OutDataTypeStr=Inherit: Same as second input  OutDataType=fixdt(1, 16)  OutScaling=2^-10  DoSatur=off
  Sum10 : Sum  Inputs=+-
  Sum11 : Sum  Inputs=+-
  Sum12 : Sum
  Sum13 : Sum  Inputs=-+
  Switch1 : Switch  Criteria=u2 ~= 0
  Switch2 : Switch  Criteria=u2 ~= 0  OutDataTypeStr=single
  Unit Delay : UnitDelay  SampleTime=-1  HasFrameUpgradeWarning=on
  Weight/N3 : Constant  Value=0.02  OutDataTypeStr=single  SampleTime=-1
  axvModeldiff : Outport
  axvModel_Ref : Outport  Port=2
  axvModelResidual : Outport  Port=3
  wires:
  Sum13/1 -> axvModel_Ref/1
  Constant/1 -> Product/2
  Constant1/1 -> Gain1/1, Saturation Dynamic/1
  axvTorqMean/1 -> Sum10/1, Sum13/2
  [t_axvModelResidual] -> Switch2/1
  Product3/1 -> Sum12/1
  Saturation Dynamic/1 -> Sum11/1
  [t_axvModelResidual] -> Product/1
  Enable/1 -> Switch1/2, Switch2/2
  Gain1/1 -> Saturation Dynamic/3
  AxRef/1 -> Sum10/2
  [axvModeldiff] -> Abs1/1
  Abs1/1 -> FilterTime/1
  Sum12/1 -> axvModelResidual/1, [t_axvModelResidual]
  Sum10/1 -> [axvModeldiff], axvModeldiff/1
  FilterTime/1 -> Product4/2
  [axvModeldiff] -> Switch1/1
  Switch2/1 -> Sum13/1, Unit Delay/1
  Product/1 -> Switch2/3
  Unit Delay/1 -> Sum11/2, Sum12/2, Switch1/3
  Product4/1 -> Product3/1
  Switch1/1 -> Saturation Dynamic/2
  Weight/N3/1 -> Product4/1
  Sum11/1 -> Product3/2

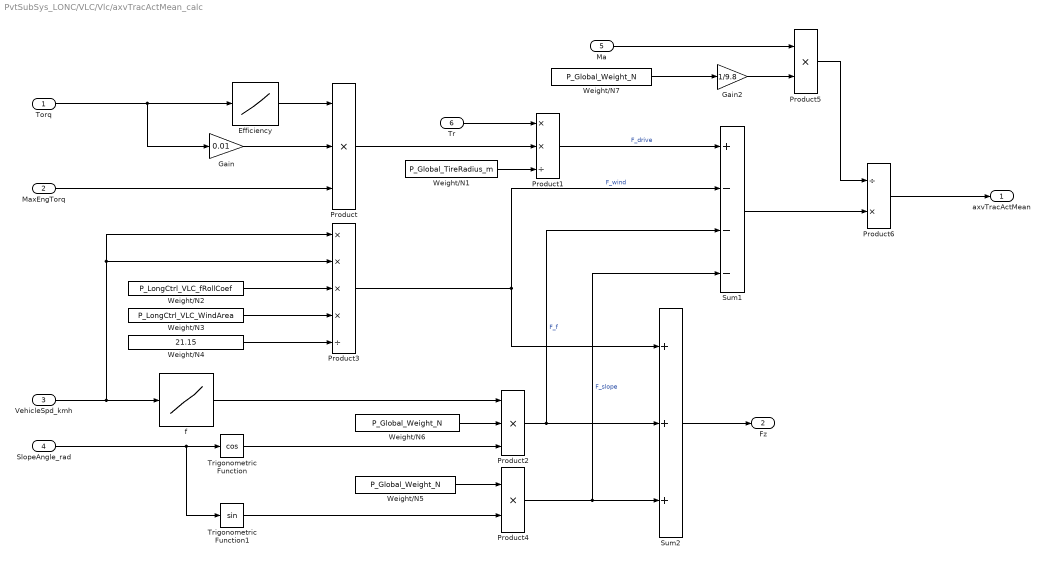
== system PvtSubSys_LONC/VLC/Vlc/axvTracActMean_calc ==
  Torq : Inport  OutDataTypeStr=single
  MaxEngTorq : Inport  Port=2  OutDataTypeStr=single
  VehicleSpd_kmh : Inport  Port=3  OutDataTypeStr=single
  SlopeAngle_rad : Inport  Port=4  OutDataTypeStr=single
  Ma : Inport  Port=5  OutDataTypeStr=single
  Tr : Inport  Port=6  OutDataTypeStr=single
  Efficiency : Lookup_n-D  NumberOfTableDimensions=1  BreakpointsForDimension1=P_LongCtrl_VLCtorqCharEngEfficientXAxis  Table=P_LongCtrl_VLCengEfficientCharYAxis  ExtrapMethod=Clip  UseLastTableValue=on  RndMeth=Simplest  InputSameDT=on
  Gain : Gain  Gain=0.01
  Gain2 : Gain  Gain=1/9.8
  Product : Product  Inputs=***  RndMeth=Zero
  Product1 : Product  Inputs=**/  RndMeth=Zero
  Product2 : Product  Inputs=***  RndMeth=Zero
  Product3 : Product  Inputs=****/  RndMeth=Zero
  Product4 : Product  Inputs=**  RndMeth=Zero
  Product5 : Product  Inputs=**  RndMeth=Zero
  Product6 : Product  Inputs=/*  RndMeth=Zero
  Sum1 : Sum  Inputs=+---
  Sum2 : Sum  Inputs=+++
  Trigonometric Function : Trigonometry  Operator=cos
  Trigonometric Function1 : Trigonometry
  Weight/N1 : Constant  Value=P_Global_TireRadius_m  OutDataTypeStr=single
  Weight/N2 : Constant  Description=0.395  Value=P_LongCtrl_VLC_fRollCoef  OutDataTypeStr=single
      settings: AttributesFormatString=%<Description>
  Weight/N3 : Constant  Description=2.4  Value=P_LongCtrl_VLC_WindArea  OutDataTypeStr=single
      settings: AttributesFormatString=%<Description>
  Weight/N4 : Constant  Value=21.15  OutDataTypeStr=single
  Weight/N5 : Constant  Value=P_Global_Weight_N  OutDataTypeStr=single
  Weight/N6 : Constant  Value=P_Global_Weight_N  OutDataTypeStr=single
  Weight/N7 : Constant  Value=P_Global_Weight_N  OutDataTypeStr=single
  f : Lookup_n-D  NumberOfTableDimensions=1  BreakpointsForDimension1=P_LongCtrl_VLCcoefFXAxis  Table=P_LongCtrl_VLCcoefFYAxis  ExtrapMethod=Clip  UseLastTableValue=on  RndMeth=Simplest  InputSameDT=on
  axvTracActMean : Outport  OutDataTypeStr=single
  Fz : Outport  Port=2  OutDataTypeStr=single
  wires:
  f/1 -> Product2/1
  Weight/N1/1 -> Product1/3
  Weight/N5/1 -> Product4/1
  Weight/N6/1 -> Product2/2
  Weight/N7/1 -> Gain2/1
  Sum2/1 -> Fz/1
  Trigonometric Function1/1 -> Product4/2
  Product6/1 -> axvTracActMean/1
  MaxEngTorq/1 -> Product/3
  Tr/1 -> Product1/1
  Ma/1 -> Product5/1
  Gain2/1 -> Product5/2
  Product5/1 -> Product6/1
  Sum1/1 -> Product6/2
  Product4/1 -> Sum1/4, Sum2/3  "F_slope"
  Product2/1 -> Sum2/2, Sum1/3  "F_f"
  Product3/1 -> Sum2/1, Sum1/2  "F_wind"
  Weight/N4/1 -> Product3/5
  Weight/N3/1 -> Product3/4
  Weight/N2/1 -> Product3/3
  Product1/1 -> Sum1/1  "F_drive"
  Trigonometric Function/1 -> Product2/3
  SlopeAngle_rad/1 -> Trigonometric Function1/1, Trigonometric Function/1
  VehicleSpd_kmh/1 -> Product3/2, Product3/1, f/1
  Product/1 -> Product1/2
  Gain/1 -> Product/2
  Efficiency/1 -> Product/1
  Torq/1 -> Gain/1, Efficiency/1

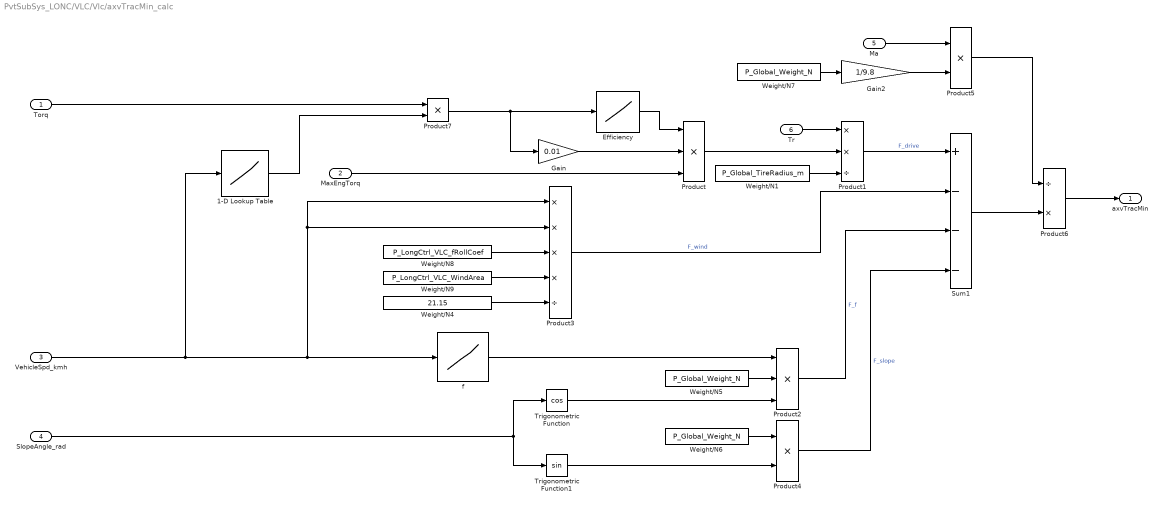
== system PvtSubSys_LONC/VLC/Vlc/axvTracMin_calc ==
  Torq : Inport
  MaxEngTorq : Inport  Port=2
  VehicleSpd_kmh : Inport  Port=3
  SlopeAngle_rad : Inport  Port=4
  Ma : Inport  Port=5
  Tr : Inport  Port=6
  1-D Lookup Table : Lookup_n-D  NumberOfTableDimensions=1  BreakpointsForDimension1=[0 10 20 30 40 50 60 70 80 90 100]  Table=[0 0 0.1 0.65 0.75 0.8 0.85 0.9 0.95 1 1]  ExtrapMethod=Clip  UseLastTableValue=on  InternalRulePriority=Speed  RndMeth=Simplest  InputSameDT=on
  Efficiency : Lookup_n-D  NumberOfTableDimensions=1  BreakpointsForDimension1=P_LongCtrl_VLCtorqCharEngEfficientXAxis  Table=P_LongCtrl_VLCengEfficientCharYAxis  ExtrapMethod=Clip  UseLastTableValue=on  RndMeth=Simplest  InputSameDT=on
  Gain : Gain  Gain=0.01
  Gain2 : Gain  Gain=1/9.8
  Product : Product  Inputs=***  RndMeth=Zero
  Product1 : Product  Inputs=**/  RndMeth=Zero
  Product2 : Product  Inputs=***  RndMeth=Zero
  Product3 : Product  Inputs=****/  RndMeth=Zero
  Product4 : Product  Inputs=**  RndMeth=Zero
  Product5 : Product  Inputs=**  RndMeth=Zero
  Product6 : Product  Inputs=/*  RndMeth=Zero
  Product7 : Product
  Sum1 : Sum  Inputs=+---
  Trigonometric Function : Trigonometry  Operator=cos
  Trigonometric Function1 : Trigonometry
  Weight/N1 : Constant  Value=P_Global_TireRadius_m  OutDataTypeStr=single
  Weight/N4 : Constant  Value=21.15  OutDataTypeStr=single
  Weight/N5 : Constant  Value=P_Global_Weight_N  OutDataTypeStr=single
  Weight/N6 : Constant  Value=P_Global_Weight_N  OutDataTypeStr=single
  Weight/N7 : Constant  Value=P_Global_Weight_N  OutDataTypeStr=single
  Weight/N8 : Constant  Description=0.395  Value=P_LongCtrl_VLC_fRollCoef  OutDataTypeStr=single
      settings: AttributesFormatString=%<Description>
  Weight/N9 : Constant  Description=2.4  Value=P_LongCtrl_VLC_WindArea  OutDataTypeStr=single
      settings: AttributesFormatString=%<Description>
  f : Lookup_n-D  NumberOfTableDimensions=1  BreakpointsForDimension1=P_LongCtrl_VLCcoefFXAxis  Table=P_LongCtrl_VLCcoefFYAxis  ExtrapMethod=Clip  UseLastTableValue=on  RndMeth=Simplest  InputSameDT=on
  axvTracMin : Outport
  wires:
  Torq/1 -> Product7/1
  1-D Lookup Table/1 -> Product7/2
  Product7/1 -> Efficiency/1, Gain/1
  Tr/1 -> Product1/1
  Ma/1 -> Product5/1
  f/1 -> Product2/1
  Weight/N1/1 -> Product1/3
  Weight/N6/1 -> Product4/1
  Weight/N5/1 -> Product2/2
  Weight/N7/1 -> Gain2/1
  Trigonometric Function1/1 -> Product4/2
  Product6/1 -> axvTracMin/1
  MaxEngTorq/1 -> Product/3
  Gain2/1 -> Product5/2
  Product5/1 -> Product6/1
  Sum1/1 -> Product6/2
  Product4/1 -> Sum1/4  "F_slope"
  Product2/1 -> Sum1/3  "F_f"
  Product3/1 -> Sum1/2  "F_wind"
  Weight/N4/1 -> Product3/5
  Weight/N9/1 -> Product3/4
  Weight/N8/1 -> Product3/3
  Product1/1 -> Sum1/1  "F_drive"
  Trigonometric Function/1 -> Product2/3
  SlopeAngle_rad/1 -> Trigonometric Function1/1, Trigonometric Function/1
  VehicleSpd_kmh/1 -> Product3/1, Product3/2, f/1, 1-D Lookup Table/1
  Product/1 -> Product1/2
  Gain/1 -> Product/2
  Efficiency/1 -> Product/1

== system PvtSubSys_LONC/VLC/Vlc/EC/LP ==
  Raw : Inport
  Constant1 : Constant  Value=0.05  OutDataTypeStr=single
  Constant3 : Constant  Value=0.02  OutDataTypeStr=single
  Product7 : Product  Inputs=*/  RndMeth=Zero
  Product8 : Product  RndMeth=Zero
  Sum14 : Sum
  Sum9 : Sum  Inputs=+-
  Unit Delay : UnitDelay  SampleTime=-1  HasFrameUpgradeWarning=on
  Out : Outport
  wires:
  Constant1/1 -> Product7/2
  Constant3/1 -> Product7/1
  Sum9/1 -> Product8/2
  Sum14/1 -> Out/1, Unit Delay/1
  Unit Delay/1 -> Sum14/2, Sum9/2
  Raw/1 -> Sum9/1
  Product8/1 -> Sum14/1
  Product7/1 -> Product8/1

== system PvtSubSys_LONC/VLC/Vlc/FF_Control/LP ==
  Raw : Inport
  tauFxvCvFilter : Inport  Port=2
  Add2 : Sum  Inputs=+-
  Add3 : Sum
  Product4 : Product  Inputs=**  RndMeth=Zero
  Unit Delay : UnitDelay  SampleTime=-1  HasFrameUpgradeWarning=on
  Out : Outport
  wires:
  tauFxvCvFilter/1 -> Product4/1
  Product4/1 -> Add3/1
  Add2/1 -> Product4/2
  Unit Delay/1 -> Add3/2, Add2/2
  Add3/1 -> Unit Delay/1, Out/1
  Raw/1 -> Add2/1

== system PvtSubSys_LONC/VLC/Vlc/FF_Control/LP1 ==
  Raw : Inport
  VxvRef : Inport  Port=2
  Constant2 : Constant  Value=0.02  OutDataTypeStr=single
  FilterTime : Lookup_n-D  NumberOfTableDimensions=1  BreakpointsForDimension1=[0,10,20,30,40]  Table=[0.5,0.5,2,3,3]  ExtrapMethod=Clip  UseLastTableValue=on  RndMeth=Simplest  InputSameDT=on
  Product2 : Product  Inputs=*/  RndMeth=Zero
  Product6 : Product  OutDataTypeStr=single  RndMeth=Zero
  Sum6 : Sum  Inputs=+-
  Sum7 : Sum
  Unit Delay : UnitDelay  SampleTime=-1  HasFrameUpgradeWarning=on
  Out : Outport
  wires:
  VxvRef/1 -> FilterTime/1
  Raw/1 -> Sum6/1
  Product6/1 -> Sum7/1
  Product2/1 -> Product6/1
  Sum6/1 -> Product6/2
  FilterTime/1 -> Product2/2
  Constant2/1 -> Product2/1
  Unit Delay/1 -> Sum6/2, Sum7/2
  Sum7/1 -> Unit Delay/1, Out/1

== system PvtSubSys_LONC/VLC/Vlc/PI_Control/If Action Subsystem ==
  In1 : Inport
  Action Port : ActionPort
  Out1 : Outport
  wires:
  In1/1 -> Out1/1

== system PvtSubSys_LONC/VLC/Vlc/PI_Control/If Action Subsystem1 ==
  In1 : Inport
  Action Port : ActionPort
  Gain2 : Gain  Gain=-1
  Out1 : Outport
  wires:
  Gain2/1 -> Out1/1
  In1/1 -> Gain2/1

== system PvtSubSys_LONC/VLC/Vlc/SwitchToBrakeMode/LP filter ==
  Raw : Inport
  FilterTime : Constant  Value=0.1  OutDataTypeStr=single
  Product1 : Product  RndMeth=Zero
  Product4 : Product  Inputs=*/  RndMeth=Zero
  Sum4 : Sum  Inputs=+-
  Sum5 : Sum
  Unit Delay : UnitDelay  SampleTime=-1  HasFrameUpgradeWarning=on
  Weight/N3 : Constant  Value=0.02  OutDataTypeStr=single
  output : Outport
  wires:
  Unit Delay/1 -> Sum4/2, Sum5/2
  Sum4/1 -> Product1/2
  Sum5/1 -> Unit Delay/1, output/1
  Product1/1 -> Sum5/1
  Raw/1 -> Sum4/1
  Weight/N3/1 -> Product4/1
  Product4/1 -> Product1/1
  FilterTime/1 -> Product4/2

== system PvtSubSys_LONC/VLC/Vlc/UpdateFlagCalc/Timer ==
  Falling : Inport
  Detect Decrease : simulink/Logic and Bit Operations/Detect Decrease  vinit=0.0  OutDataTypeStr=uint8
  MATLAB Function : MATLAB Function  TreatAsAtomicUnit=on
  Unit Delay : UnitDelay  SampleTime=-1  HasFrameUpgradeWarning=on
  Unit Delay1 : UnitDelay  SampleTime=-1  HasFrameUpgradeWarning=on
  Timer : Outport
  wires:
  Unit Delay/1 -> MATLAB Function/3(StartTimerK1)
  Detect Decrease/1 -> MATLAB Function/1(Falling)
  Unit Delay1/1 -> MATLAB Function/2(TimerK1)
  MATLAB Function/2(StartTimer) -> Unit Delay/1
  Falling/1 -> Detect Decrease/1
  MATLAB Function/1(Timer) -> Unit Delay1/1, Timer/1

== system PvtSubSys_LONC/VLC/Vlc/axvClosedLoopControlCalc/LP1 ==
  Raw : Inport
  Constant3 : Constant  Value=0.02  OutDataTypeStr=single
  FilterTime2 : Constant  Value=0.1  OutDataTypeStr=single
  Product7 : Product  Inputs=*/  RndMeth=Zero
  Product8 : Product  RndMeth=Zero
  Sum14 : Sum
  Sum9 : Sum  Inputs=+-
  Unit Delay : UnitDelay  SampleTime=-1  HasFrameUpgradeWarning=on
  Out : Outport
  wires:
  Constant3/1 -> Product7/1
  FilterTime2/1 -> Product7/2
  Sum9/1 -> Product8/2
  Sum14/1 -> Unit Delay/1, Out/1
  Unit Delay/1 -> Sum9/2, Sum14/2
  Raw/1 -> Sum9/1
  Product8/1 -> Sum14/1
  Product7/1 -> Product8/1

== matlab function PvtSubSys_LONC/VLC/Vlc/Subsystem/MATLAB Function ==
  data: u input; ACCModeSts output; Counter input single; CounterK1 output single
function [ACCModeSts,CounterK1] = fcn(u,Counter)
if (u(1)==7)&&((u(2)==6)||u(2)==(9))
    Counter=single(76);
end
if Counter>0
    ACCModeSts=uint8(6);
    CounterK1=max(single(0),Counter-single(1));
else
    ACCModeSts = u(1);
    CounterK1=single(0);
end

== stateflow chart PvtSubSys_LONC/VLC/Vlc/DC/StandstillAccel2 ==
  (default) -> (junction 44)
  (junction 44) -> (junction 48) [order 1] : [(VLCState==3)]
  (junction 44) -> (junction 46) [order 2] : {SlidTimer = single(0);
      | VlcSlidAxTar = VlcAxTar;}
  (junction 48) -> (junction 49) : {SlidTimer=min(single(100),SlidTimer+single(1));
      | SlidAx = min(single(-0.3),VlcAxTar);
      | VlcSlidAxTar = max(accelSlidHold,(SlidAx+jerkSlidHold*tCycle*SlidTimer));}
  (junction 49) -> (junction 46)
  (junction 46) -> (junction 1)
  (junction 1) -> (junction 3) [order 1] : [ACCmode(1)==6||ACCmode(1)==9]
  (junction 1) -> (junction 7) [order 2] : {timer=single(0);
      | decelReq=VlcSlidAxTar;}
  (junction 3) -> (junction 5) : {timer=min(single(100),timer+single(1));
      |  Ax=min(single(-0.3),VlcAxTar);
      | decelReq=max(accelHoldMin,(Ax+jerkHold*tCycle*timer));}
  (junction 5) -> (junction 7)
  (junction 7) -> (junction 14)
  (junction 14) -> (junction 19) [order 1] : [(ACCmode(2)==6||ACCmode(2)==9)&&(ACCmode(1)==7)]
  (junction 14) -> (junction 23) [order 2] : {timerFailure=max(uint8(0),timerFailure-uint8(1));}
  (junction 19) -> (junction 21) : {timerFailure=uint8(75);}
  (junction 21) -> (junction 23)
  (junction 23) -> (junction 26)
  (junction 26) -> (junction 28) [order 1] : [timerFailure>0]
  (junction 26) -> (junction 32) [order 2] : {decelReqActive=false;}
  (junction 28) -> (junction 30) : {decelReq=decelReqK1;
      |  decelReqActive=true;}
  (junction 30) -> (junction 32)
  (junction 32) -> (junction 35) : {decelReqK1=decelReq;}
  data: decelReqActive output; VlcAxTar input single; ACCmode input; timer local single =single(0); decelReq output single; Ax local; accelHoldMin input; jerkHold input single; timerFailure local =uint8(0); decelReqK1 local; tCycle input; VLCState input; accelSlidHold input; jerkSlidHold input; SlidAx local; VlcSlidAxTar local; SlidTimer local

== matlab function PvtSubSys_LONC/VLC/Vlc/EC/FxLimit ==
  data: tEC input single; Up output single; UpDelta input single; VxvRef input single; LowDelta input single; DCK1 input boolean; EC input boolean; Driveoff input boolean; VLCState input; tECDC input; CounterK1 input single; Low output single; Counter output single; Counter2K1 input single; Counter2 output single; P_LongCtrl_VLCCounterDrvOff2EC parameter single; P_LongCtrl_VLCCounterDC2ECTorqDelay parameter single; P_LongCtrl_VLCUpperJerkCounterDrvOff2EC parameter single; P_LongCtrl_VLCLowerJerkCounterDrvOff2EC parameter single
function [Up,Low,Counter,Counter2] = fcn(tEC,UpDelta,VxvRef,LowDelta,DCK1,EC,Driveoff,VLCState,tECDC,CounterK1,Counter2K1, P_LongCtrl_VLCCounterDrvOff2EC, P_LongCtrl_VLCCounterDC2ECTorqDelay, P_LongCtrl_VLCUpperJerkCounterDrvOff2EC, P_LongCtrl_VLCLowerJerkCounterDrvOff2EC)
%#codegen
if VLCState==3
    Up = min(tECDC*0.5,UpDelta);
    Low = max(-tECDC,LowDelta);
    Counter = single(0);
    Counter2 = single(0);
else
    Counter = single(max(CounterK1-1,single(0))); 
    Counter2 = single(max(Counter2K1-1,single(0))); 
    if ((Driveoff(1)==1)&&(Driveoff(2)==0))
        Counter=P_LongCtrl_VLCCounterDrvOff2EC;             
    else
        if (VxvRef>0.3)&&(EC(1)==1)&&(DCK1==1)
            Counter2=P_LongCtrl_VLCCounterDC2ECTorqDelay;         
        end
    end
    if ( Counter>0)
        Up=P_LongCtrl_VLCUpperJerkCounterDrvOff2EC;
        Low=P_LongCtrl_VLCLowerJerkCounterDrvOff2EC;
    else
        Up = min(tEC*single(0.5),UpDelta);
        Low = max(-tEC, LowDelta);
        if Counter2>0
            Up = min(tEC*single(0.1),UpDelta);
        end
    end
end

== matlab function PvtSubSys_LONC/VLC/Vlc/EC/MATLAB Function ==
  data: EngTorq_k1 input; NetEngTorq input; y output; EC_enable_k1 input
function y = fcn(EngTorq_k1,NetEngTorq,EC_enable_k1)
%#codegen
if EC_enable_k1==0
    y = NetEngTorq;
else
    y = EngTorq_k1;
end
